simulink model "FM"  (R2020b)
settings: Solver=VariableStepAuto  StartTime=0.0  StopTime=10.0  RelTol=1e-3
libraries: dsparch4 x1, commsynccomp2 x1, dspsigops x1
settings Model: Creator=htn  LastModifiedBy=htn

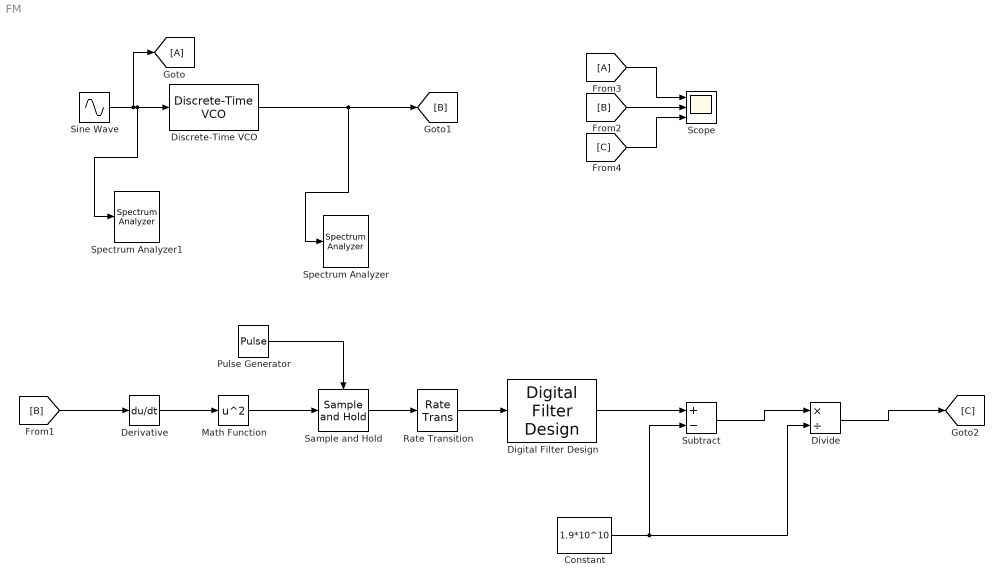
== system FM ==
  Constant : Constant  Value=1.9*10^10
  Derivative : Derivative
  Digital Filter Design : dsparch4/Digital Filter Design  mwdsp_browser_bugfix_var=off
  Discrete-Time VCO : commsynccomp2/Discrete-Time VCO  Ac=5  Fc=3000  Kc=2000  Ph=0  ts=1/20000
      settings: SourceProductBaseCode=CM
  Divide : Product  Inputs=*/
  Math Function : Math  Operator=square  SaturateOnIntegerOverflow=on
  Pulse Generator : DiscretePulseGenerator  PulseType=Time based  Period=1/20000  PulseWidth=50
  Rate Transition : RateTransition  OutPortSampleTime=1/20000
  Sample and Hold : dspsigops/Sample and Hold  trig=Rising edge  initCond=0  latchinput=off
  Scope : Scope  NumInputPorts=3
  Sine Wave : Sin  Frequency=2*pi*500  SampleTime=1/20000
  Spectrum Analyzer : SpectrumAnalyzer
  Spectrum Analyzer1 : SpectrumAnalyzer
  Subtract : Sum  Inputs=+-
  wires:
  Sine Wave/1 -> [A], Spectrum Analyzer1/1, Discrete-Time VCO/1
  Discrete-Time VCO/1 -> Spectrum Analyzer/1, [B]
  [B] -> Derivative/1
  Derivative/1 -> Math Function/1
  Math Function/1 -> Sample and Hold/1
  Pulse Generator/1 -> Sample and Hold/Trigger
  Sample and Hold/1 -> Rate Transition/1
  Rate Transition/1 -> Digital Filter Design/1
  [B] -> Scope/2
  [A] -> Scope/1
  [C] -> Scope/3
  Digital Filter Design/1 -> Subtract/1
  Subtract/1 -> Divide/1
  Divide/1 -> [C]
  Constant/1 -> Divide/2, Subtract/2
